simulink subsystem "AS5600_Sensor"  (R2022b)
settings: Solver=VariableStepAuto  StartTime=0.0  StopTime=10.0  RelTol=1e-3
model mask{sensor_model=0.5, wrapping=on, offset=0}
  mask prompts: sensor_model "Sensor Parameters struct:"; wrapping "Angle wrapping:"; offset "Magnet Alignment Error [mm]:"
settings Model: Creator=gotta  LastModifiedBy=gotta

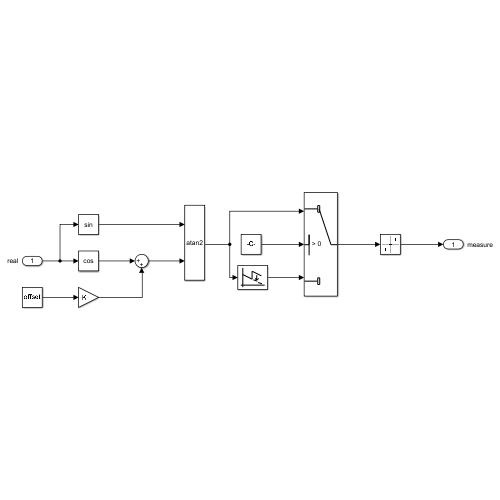
[thumbnail: Simulink's stored preview of the top-level diagram]
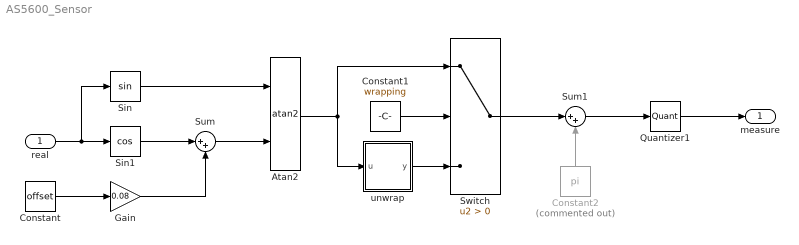
== system AS5600_Sensor ==
  real : Inport
  Atan2 : Trigonometry  Operator=atan2
  Constant : Constant  Value=offset
  Constant1 : Constant  Value=wrapping
  Constant2 : Constant  Commented=on  Value=pi
  Gain : Gain  Gain=0.08
  Quantizer1 : Quantizer  QuantizationInterval=sensor_model.Astep
  Sin : Trigonometry
  Sin1 : Trigonometry  Operator=cos
  Sum : Sum  Inputs=|++
  Sum1 : Sum  Inputs=|++
  Switch : Switch  Criteria=u2 > Threshold  SaturateOnIntegerOverflow=off  InputSameDT=off
  unwrap : Subsystem
  measure : Outport
  wires:
  Constant2/1 -> Sum1/2
  Sum1/1 -> Quantizer1/1
  real/1 -> Sin1/1, Sin/1
  Gain/1 -> Sum/2
  Constant1/1 -> Switch/2
  Quantizer1/1 -> measure/1
  Switch/1 -> Sum1/1
  unwrap/1(y) -> Switch/3
  Atan2/1 -> Switch/1, unwrap/1(u)
  Sin/1 -> Atan2/1
  Sum/1 -> Atan2/2
  Constant/1 -> Gain/1
  Sin1/1 -> Sum/1

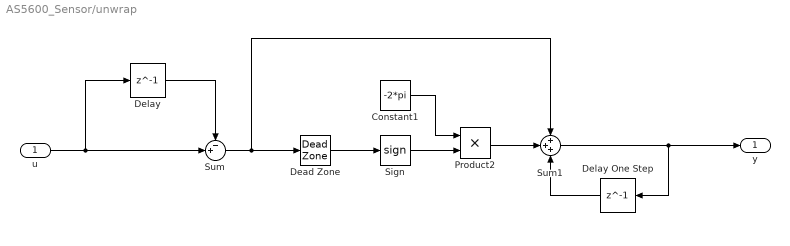
== system AS5600_Sensor/unwrap ==
  u : Inport
  Constant1 : Constant  Value=-2*pi
  Dead Zone : DeadZone  LowerValue=-pi  UpperValue=pi
  Delay : Delay  DelayLength=1
  Delay One Step : Delay  DelayLength=1
  Product2 : Product
  Sign : Signum
  Sum : Sum  Inputs=-+|
  Sum1 : Sum  Inputs=+++
  y : Outport
  wires:
  Delay One Step/1 -> Sum1/3
  Sum1/1 -> y/1, Delay One Step/1
  Product2/1 -> Sum1/2
  Constant1/1 -> Product2/1
  Sign/1 -> Product2/2
  Dead Zone/1 -> Sign/1
  Sum/1 -> Sum1/1, Dead Zone/1
  Delay/1 -> Sum/1
  u/1 -> Sum/2, Delay/1
